simulink model "Rocky"  (R2021b)
settings: Solver=VariableStepAuto  StartTime=0.0  StopTime=10.0  RelTol=1e-3
undefined symbols (not defined in the file): a, b, Ci, Cp, g, Ji, Jp, Ki, Kp, l
settings Model: Creator=atan  LastModifiedBy=mluser
settings SolverCC: AlgebraicLoopSolver=TrustRegion
settings DebuggingCC: SFMachineParentedDataDiag=warning

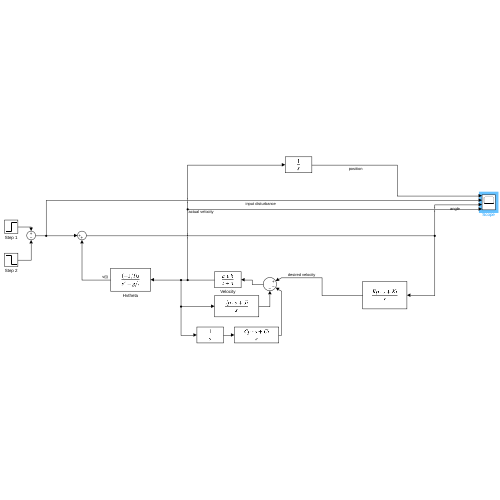
[thumbnail: Simulink's stored preview of the top-level diagram]
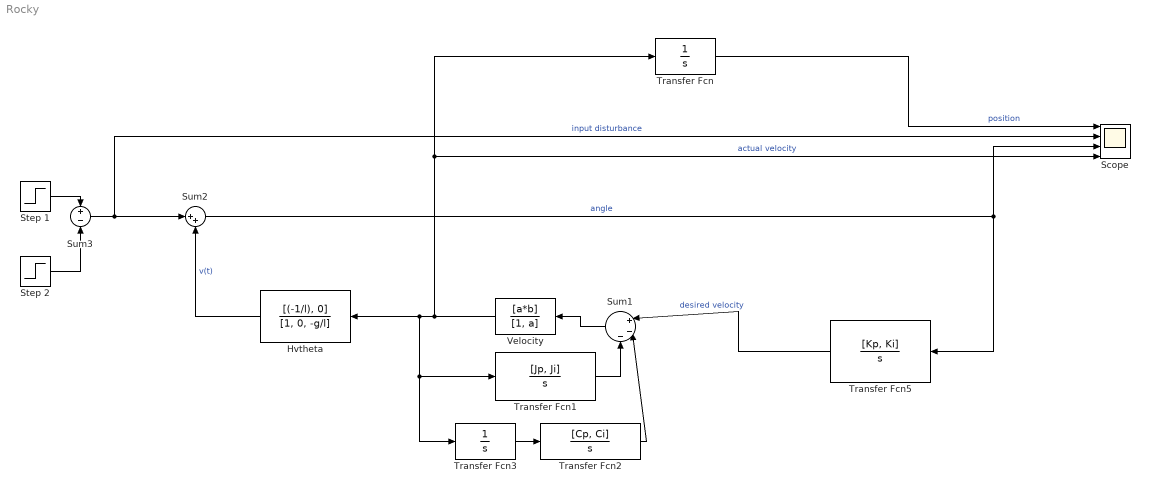
== system Rocky ==
  Hvtheta : TransferFcn  Numerator=[(-1/l), 0]  Denominator=[1, 0, -g/l]
  Scope : Scope  NumInputPorts=4
  Step 1 : Step  Time=0.025  SampleTime=0
  Step 2 : Step  Time=0.050  After=-1  SampleTime=0
  Sum1 : Sum  Inputs=|+--
  Sum2 : Sum  Inputs=|++
  Sum3 : Sum  Inputs=+-
  Transfer Fcn : TransferFcn  Denominator=[ 1 0]
  Transfer Fcn1 : TransferFcn  Numerator=[Jp, Ji]  Denominator=[1 0]
  Transfer Fcn2 : TransferFcn  Numerator=[Cp, Ci]  Denominator=[1 , 0]
  Transfer Fcn3 : TransferFcn  Denominator=[1 0]
  Transfer Fcn5 : TransferFcn  Numerator=[Kp, Ki]  Denominator=[1 0]
  Velocity : TransferFcn  Numerator=[a*b]  Denominator=[1, a]
  wires:
  Velocity/1 -> Transfer Fcn3/1, Transfer Fcn1/1, Hvtheta/1, Transfer Fcn/1, Scope/4  "actual velocity"
  Sum1/1 -> Velocity/1
  Transfer Fcn1/1 -> Sum1/3
  Transfer Fcn2/1 -> Sum1/2
  Transfer Fcn5/1 -> Sum1/1  "desired velocity"
  Hvtheta/1 -> Sum2/2  "v(t)"
  Sum2/1 -> Scope/3, Transfer Fcn5/1  "angle"
  Step 1/1 -> Sum3/1
  Step 2/1 -> Sum3/2
  Sum3/1 -> Scope/2, Sum2/1  "input disturbance"
  Transfer Fcn/1 -> Scope/1  "position"
  Transfer Fcn3/1 -> Transfer Fcn2/1
